simulink model "noisy_step_v_RL_circuit"  (R2017b)
settings: Solver=VariableStepAuto  StartTime=0.0  StopTime=simTime  RelTol=1e-3
values from neighbouring files (symbols this model uses):
  L = 3    [RL_circuit_data_generator.m]    (also in RL_circuit_data_generator_2.m; gera_dados_circuitoRL.m = 0.001; multi_pinn_data_generation.m)
  noisePower = 1e-6    (= 1e-06)    [RL_circuit_data_generator.m]    (also in RL_circuit_data_generator_2.m)
  R = 3    [RL_circuit_data_generator.m]    (also in RL_circuit_data_generator_2.m; gera_dados_circuitoRL.m = 1000; multi_pinn_data_generation.m)
  simStepSize = 1e-2    (= 0.01)    [RL_circuit_data_generator.m]    (also in RL_circuit_data_generator_2.m; multi_pinn_data_generation.m)
  v0 = j    [RL_circuit_data_generator_2.m]    (also in multi_pinn_data_generation.m = 0)
libraries: simulink x1
settings Model: Creator=Eduardo Rehbein  LastModifiedBy=Eduardo

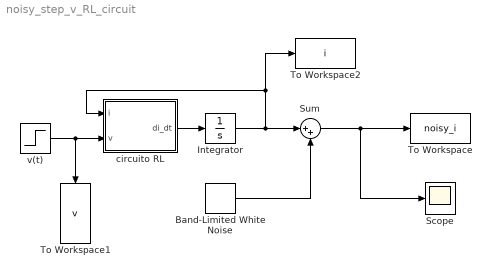
== system noisy_step_v_RL_circuit ==
  Band-Limited White Noise : simulink/Sources/Band-Limited White Noise  Cov=[noisePower]  Ts=simStepSize  seed=[23341]
  Integrator : Integrator
  Scope : Scope
  Sum : Sum  Inputs=|++
  To Workspace : ToWorkspace  VariableName=noisy_i  SaveFormat=Timeseries  SampleTime=-1
  To Workspace1 : ToWorkspace  VariableName=v  SaveFormat=Timeseries  SampleTime=-1
  To Workspace2 : ToWorkspace  VariableName=i  SaveFormat=Timeseries  SampleTime=-1
  circuito RL : MATLAB Function  TreatAsAtomicUnit=on
  v(t) : Step  Time=0  After=v0  SampleTime=0
  wires:
  circuito RL/1(di_dt) -> Integrator/1
  v(t)/1 -> circuito RL/2(v), To Workspace1/1
  Band-Limited White Noise/1 -> Sum/2
  Integrator/1 -> To Workspace2/1, circuito RL/1(i), Sum/1
  Sum/1 -> To Workspace/1, Scope/1

== matlab function noisy_step_v_RL_circuit/circuito RL ==
  settings: updateMethod=DISCRETE  sampleTime=simStepSize
  data: i input; di_dt output; v input; R parameter; L parameter
function di_dt = fcn(i, v, R, L)

di_dt = (1/L)*(v - R*i);
